simulink model "CSTR_ol"  (R2025b)
settings: Solver=ode15s  StartTime=0.0  StopTime=20  RelTol=1e-7  AbsTol=1e-7  EnableMultiTasking=on
InitFcn:
  | data_CSTR
undefined symbols (not defined in the file or in its folder): cbar_sim, cfbar_sim, cp, cstrfun, DH, ER, ko, q, rho, Tbar_sim, Tcbar_sim, Tf, UA, V
libraries: simulink x1
settings Model: ExtModeTrigMode=oneshot  ExtModeArmWhenConnect=off  Creator=scattolini  LastModifiedBy=seby
settings SolverCC: AutoScaleAbsTol=off  AlgebraicLoopSolver=TrustRegion
settings DataIOCC: SaveFormat=Array  SignalLoggingSaveFormat=ModelDataLogs  SignalLoggingName=sigsOut
settings OptimizationCC: BlockReduction=off  BooleanDataType=off  DefaultParameterBehavior=Inlined  BufferReuse=off  ExpressionDepthLimit=2147483647.0  InitFltsAndDblsToZero=on  LifeSpan=inf
settings DebuggingCC: SaveWithParameterizedLinksMsg=none  UnderspecifiedInitializationDetection=Classic  MergeDetectMultiDrivingBlocksExec=none  SignalResolutionControl=TryResolveAllWithWarning  MultiTaskDSMMsg=warning  MultiTaskCondExecSysMsg=none  FcnCallInpInsideContextMsg=warning  UnconnectedInputMsg=warning  UnconnectedOutputMsg=warning  UnconnectedLineMsg=warning  StateNameClashWarn=warning  SFUnexpectedBacktrackingDiag=warning  SFNoUnconditionalDefaultTransitionDiag=warning  SFExecutionAtInitializationDiag=none  ArithmeticOperatorsInVariantConditions=warning
settings HardwareCC: ProdBitPerPointer=32.0  ProdBitPerSizeT=32.0  ProdBitPerPtrDiffT=32.0  ProdLargestAtomicFloat=None  ProdIntDivRoundTo=Undefined  ProdEndianess=Unspecified  ProdWordSize=32.0  ProdHWDeviceType=32-bit Generic  TargetUnknown=on
settings ModelReferenceCC: EnableRefExpFcnMdlSchedulingChecks=on  PropagateSignalLabelsOutOfModel=off
settings SFSimCC: SimUseLocalCustomCode=off  CustomCodeUndefinedFunction=UseInterfaceOnly
settings RTWCC: RTWUseLocalCustomCode=off  GPUComputeCapability=3.5
settings CodeAppCC: StateflowObjectComments=on
settings GRTTargetCC: TargetFcnLib=ansi_tfl_tmw.mat  TargetLangStandard=C89/C90 (ANSI)  CombineOutputUpdateFcns=off  GRTInterface=on
settings ConfigComp: CovMetricSettings=dw  CovSaveCumulativeToWorkspaceVar=on  CovSaveSingleToWorkspaceVar=on  CovExternalEMLEnable=off  CovSFcnEnable=off

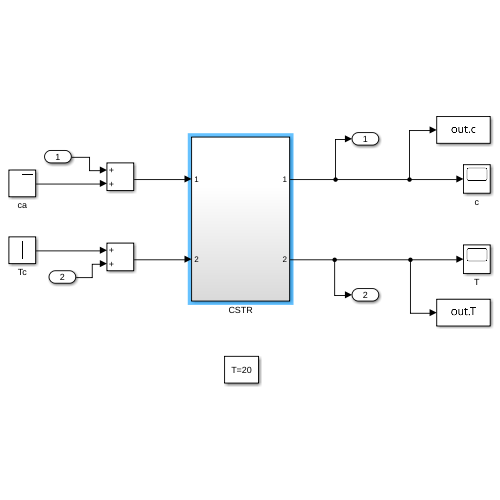
[thumbnail: Simulink's stored preview of the top-level diagram]
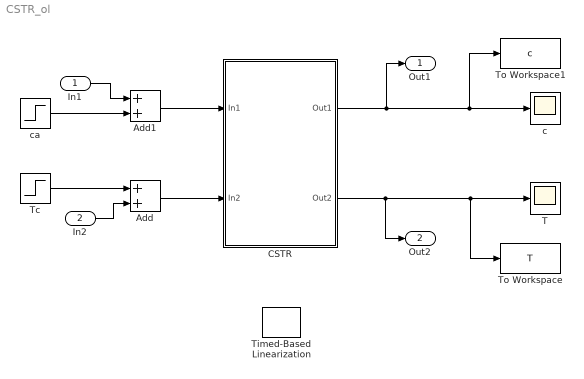
== system CSTR_ol ==
  In1 : Inport
  In2 : Inport  Port=2
  Add : Sum
  Add1 : Sum
  CSTR : Subsystem
  T : Scope
      settings: ActiveDisplayYMinimum=324.69659626194789  ActiveDisplayYMaximum=324.69659626394235
  Tc : Step  Time=0  After=Tcbar_sim  SampleTime=0
  Timed-Based Linearization : simulink/Model-Wide Utilities/Timed-Based Linearization  LinearizationTime=20  SampleTime=0
  To Workspace : ToWorkspace  VariableName=T  SaveFormat=Timeseries  SampleTime=-1
  To Workspace1 : ToWorkspace  VariableName=c  SaveFormat=Timeseries  SampleTime=-1
  c : Scope
      settings: ActiveDisplayYMinimum=0.88398396702008353  ActiveDisplayYMaximum=0.883983967020917
  ca : Step  Time=0  After=cfbar_sim  SampleTime=0
  Out1 : Outport
  Out2 : Outport  Port=2
  wires:
  CSTR/1(Out1) -> Out1/1, c/1, To Workspace1/1
  CSTR/2(Out2) -> Out2/1, T/1, To Workspace/1
  Add/1 -> CSTR/2(In2)
  Tc/1 -> Add/1
  Add1/1 -> CSTR/1(In1)
  ca/1 -> Add1/2
  In1/1 -> Add1/1
  In2/1 -> Add/2

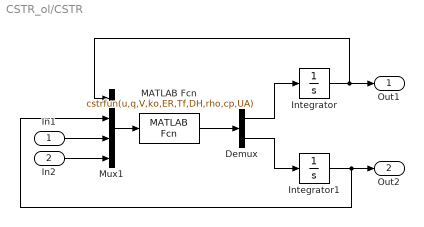
== system CSTR_ol/CSTR ==
  In1 : Inport
  In2 : Inport  Port=2
  Demux : Demux  Outputs=2
      settings: DisplayOption=none
  Integrator : Integrator  InitialCondition=cbar_sim
  Integrator1 : Integrator  InitialCondition=Tbar_sim
  MATLAB Fcn : MATLABFcn  MATLABFcn=cstrfun(u,q,V,ko,ER,Tf,DH,rho,cp,UA)
  Mux1 : Mux
  Out1 : Outport
  Out2 : Outport  Port=2
  wires:
  Mux1/1 -> MATLAB Fcn/1
  MATLAB Fcn/1 -> Demux/1
  Demux/1 -> Integrator/1
  Demux/2 -> Integrator1/1
  Integrator1/1 -> Mux1/2, Out2/1
  Integrator/1 -> Mux1/1, Out1/1
  In1/1 -> Mux1/3
  In2/1 -> Mux1/4
